simulink model "q_cal_maglev"  (Simulink 7.7)
settings: Solver=ode1  StartTime=0.0  StopTime=inf  FixedStep=0.002  RelTol=1e-3  AbsTol=1e-6
undefined symbols (not defined in the file or in its folder): HIL, qc_get_step_size
libraries: quarc_library x3, simulink x1
CloseFcn:
  | rtwprivate ssgencode ModelCloseRequest q_cal_maglev
settings Model: Creator=MLevis  LastModifiedBy=MLevis  SimulationMode=external  ExtModeTrigDuration=10000  ExtModeAutoUpdateStatusClock=off  BufferReuse=off
settings SolverCC: PositivePriorityOrder=on
settings DataIOCC: LimitDataPoints=off
settings OptimizationCC: BooleanDataType=off  InlineInvariantSignals=on  OptimizeBlockIOStorage=off  BufferReuse=off  ExpressionFolding=off  FoldNonRolledExpr=off  LocalBlockOutputs=off  InitFltsAndDblsToZero=on
settings DebuggingCC: SaveWithParameterizedLinksMsg=none  SignalResolutionControl=TryResolveAllWithWarning  SolverPrmCheckMsg=none  MultiTaskDSMMsg=warning  MultiTaskCondExecSysMsg=none  StrictBusMsg=None
settings HardwareCC: TargetHWDeviceType=32-bit Generic
settings RTWCC: SystemTargetFile=quarc_win64.tlc  TemplateMakefile=quarc_default_tmf  Description=QUARC Win64 Target  ProcessScript=quarc_win64_make_rtw_hook  IncludeERTFirstTime=on
settings STFCustomTargetCC: TargetPreCompLibLocation=C:\PROGRA~3\QUARC\lib\2011a\win64\release  FunctionExecutionProfile=off  GeneratePreprocessorConditionals=Disable all  SystemTargetFile=quarc_win64.tlc
settings GRTTargetCC: TargetPreCompLibLocation=C:\PROGRA~3\QUARC\lib\2011a\win64\release  ParMdlRefBuildCompliant=off  CompOptLevelCompliant=off  MatFileLogging=off  ExtMode=on  ExtModeMexFile=quarc_comm

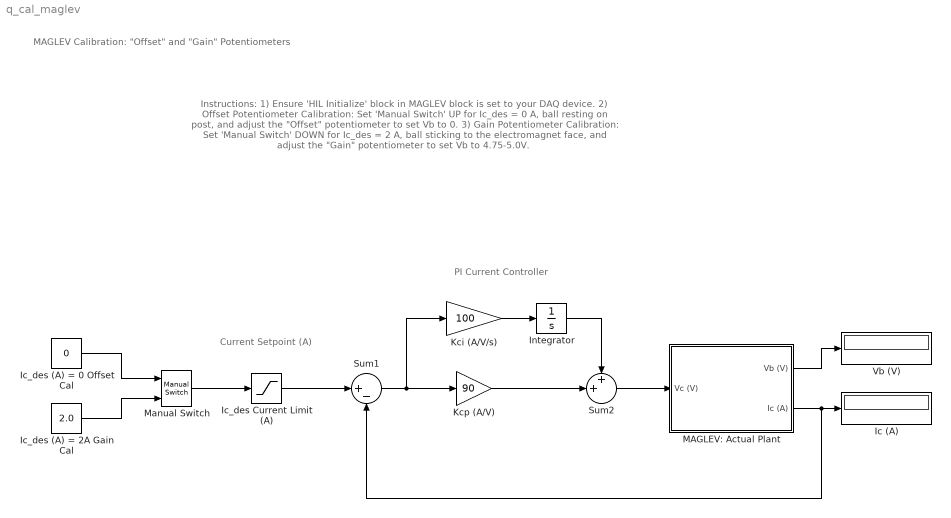
== system q_cal_maglev ==
  note: Current Setpoint (A)
  note: MAGLEV Calibration:
      | "Offset" and "Gain" Potentiometers
  note: PI Current Controller
  note: Instructions:
      | 1) Ensure 'HIL Initialize' block in MAGLEV block is set to your DAQ device.
      | 2) Offset Potentiometer Calibration:
      |       Set 'Manual Switch' UP for Ic_des = 0 A,
      |       ball resting on post, and
      |       adjust the "Offset" potentiometer to set Vb to 0.
      | 3) Gain Potentiometer Calibration:
      |       Set 'Manual Switch' DOWN for Ic_des = 2 A,
      |       ball sticking to the electromagnet face, and
      |       adjust the "Gain" potentiometer to set Vb to 4.75-5.0V.
  Ic (A) : Display
      settings: Decimation=100
  Ic_des (A) = 0 Offset Cal : Constant  Value=0
  Ic_des (A) = 2A Gain Cal : Constant  Value=2.0
  Ic_des Current Limit (A) : Saturate  UpperLimit=3  LowerLimit=- 3
  Integrator : Integrator  LimitOutput=on  UpperSaturationLimit=24  LowerSaturationLimit=-24
  Kci (A/V/s) : Gain  Gain=100  SaturateOnIntegerOverflow=on  OutDataTypeStr=Inherit: Same as input  ParamDataTypeStr=Inherit: Same as input
  Kcp (A/V) : Gain  Gain=90  SaturateOnIntegerOverflow=on  OutDataTypeStr=Inherit: Same as input  ParamDataTypeStr=Inherit: Same as input
  MAGLEV: Actual Plant : Subsystem
  Manual Switch : simulink/Signal Routing/Manual Switch  SystemSampleTime=-1  sw=1  action=0  varsize=off
  Sum1 : Sum  Inputs=|+-  SaturateOnIntegerOverflow=on  InputSameDT=on  OutDataTypeStr=Inherit: Same as first input
  Sum2 : Sum  Inputs=++|  SaturateOnIntegerOverflow=on  InputSameDT=on  OutDataTypeStr=Inherit: Same as first input
  Vb (V) : Display
      settings: Decimation=100
  wires:
  Sum1/1 -> Kcp (A/V)/1, Kci (A/V/s)/1
  Manual Switch/1 -> Ic_des Current Limit (A)/1
  MAGLEV: Actual Plant/2(Ic (A)) -> Sum1/2, Ic (A)/1
  Ic_des (A) = 2A Gain Cal/1 -> Manual Switch/2
  Ic_des Current Limit (A)/1 -> Sum1/1
  MAGLEV: Actual Plant/1(Vb (V)) -> Vb (V)/1
  Kci (A/V/s)/1 -> Integrator/1
  Kcp (A/V)/1 -> Sum2/2
  Sum2/1 -> MAGLEV: Actual Plant/1(Vc (V))
  Integrator/1 -> Sum2/1
  Ic_des (A) = 0 Offset Cal/1 -> Manual Switch/1

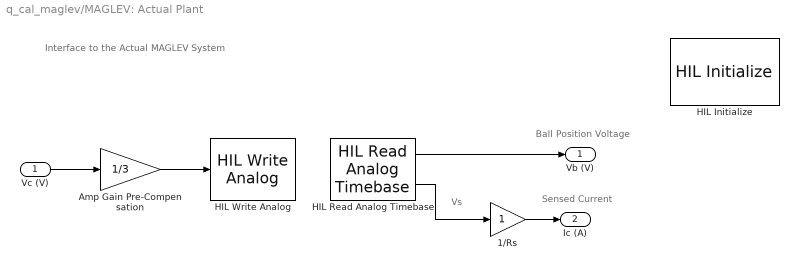
== system q_cal_maglev/MAGLEV: Actual Plant ==
  note: Interface to the Actual
      | MAGLEV System
  note: Ball Position Voltage
  note: Sensed Current
  note: Vs
  Vc (V) : Inport
  1/Rs : Gain  SaturateOnIntegerOverflow=on  OutDataTypeStr=Inherit: Same as input  ParamDataTypeStr=Inherit: Same as input
  Amp Gain Pre-Compensation : Gain  Gain=1/3  SaturateOnIntegerOverflow=on  OutDataTypeStr=Inherit: Same as input  ParamDataTypeStr=Inherit: Same as input
  HIL Initialize : quarc_library/Data Acquisition/Generic/Configuration/HIL Initialize  object_name=HIL-1  board_type=q2_usb  board_number=0  board_options=d0=digital;d1=digital;led=auto;update_rate=normal  exclusive=off  active=on  hardware_clocks=[0:2]  clock_modes=[]  initial_clock_frequencies=[]  set_clock_params_at_start=off  set_clock_params_at_switch_in=off  set_clock_frequencies_at_start=off  set_clock_frequencies_at_switch_in=off  analog_input_channels=[0:1]  analog_input_maximums=10  analog_input_minimums=-10  set_analog_input_params_at_start=on  set_analog_input_params_at_switch_in=off  analog_output_channels=[0:1]  analog_output_maximums=10  analog_output_minimums=-10  initial_analog_outputs=[0]  final_analog_outputs=[0]  watchdog_analog_outputs=0  set_analog_output_params_at_start=on  set_analog_output_params_at_switch_in=off  set_analog_outputs_at_start=on  set_analog_outputs_at_switch_in=off  set_analog_outputs_at_terminate=on  set_analog_outputs_at_switch_out=off  set_analog_outputs_on_watchdog=off  digital_input_channels=[]  digital_output_channels=[]  digital_output_configuration=[]  initial_digital_outputs=[1]  final_digital_outputs=[1]  watchdog_digital_outputs=[1]  set_digital_output_params_at_start=off  set_digital_output_params_at_switch_in=off  set_digital_outputs_at_start=on  set_digital_outputs_at_switch_in=off  set_digital_outputs_at_terminate=on  set_digital_outputs_at_switch_out=off  set_digital_outputs_on_watchdog=off  encoder_channels=[0:1]  quadrature=[4]  encoder_filter_frequency=[]  initial_encoder_counts=[0]  set_encoder_params_at_start=on  set_encoder_params_at_switch_in=off  set_encoder_counts_at_start=on  set_encoder_counts_at_switch_in=off  pwm_channels=[]  pwm_modes=[0]  pwm_frequency=1/0.020  pwm_configuration=[]  pwm_alignment=[]  pwm_polarity=[]  pwm_leading_deadband=[]  pwm_trailing_deadband=[]  initial_pwm_outputs=[0]  final_pwm_outputs=[0]  watchdog_pwm_outputs=[0]  set_pwm_params_at_start=on  set_pwm_params_at_switch_in=off  set_pwm_outputs_at_start=on  set_pwm_outputs_at_switch_in=off  set_pwm_outputs_at_terminate=on  set_pwm_outputs_at_switch_out=off  set_pwm_outputs_on_watchdog=off  other_output_channels=[]  initial_other_outputs=[]  final_other_outputs=[]  watchdog_other_outputs=[]  set_other_outputs_at_start=off  set_other_outputs_at_switch_in=off  set_other_outputs_at_terminate=off  set_other_outputs_at_switch_out=off  set_other_outputs_on_watchdog=off
  HIL Read Analog Timebase : quarc_library/Data Acquisition/Generic/Timebases/HIL Read Analog Timebase  object_name=HIL-1  clock=0  channels=[0,1]  samples_in_buffer=max(ceil(1/qc_get_step_size), 1)  active=on  vector_output=off
      settings: AttributesFormatString=(%<object_name>)
  HIL Write Analog : quarc_library/Data Acquisition/Generic/Immediate I//O/HIL Write Analog  object_name=HIL-1  channels=0  sample_time=-1  active=off  vector_input=off
  Vb (V) : Outport  InitialOutput=0
  Ic (A) : Outport  Port=2  InitialOutput=0
  wires:
  Amp Gain Pre-Compensation/1 -> HIL Write Analog/1
  Vc (V)/1 -> Amp Gain Pre-Compensation/1
  HIL Read Analog Timebase/1 -> Vb (V)/1
  HIL Read Analog Timebase/2 -> 1/Rs/1
  1/Rs/1 -> Ic (A)/1
